simulink model "Aula02_ex01"  (Simulink 7.7)
settings: Solver=VariableStepDiscrete  StartTime=0.0  StopTime=0.006  RelTol=1e-3
settings Model: Creator=Andréa  LastModifiedBy=Andréa
settings SimEventsCC: propDiagAttribOutput=1  propDiagFcnCallOutput=1  propDiagStatOutput=0

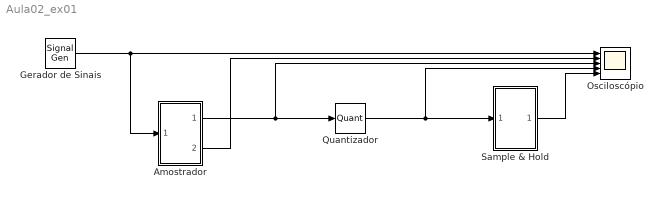
== system Aula02_ex01 ==
  Amostrador : Subsystem
  Gerador de Sinais : SignalGenerator  Frequency=500
  Osciloscópio : Scope  NumInputPorts=5
      settings: YMin=-1~-1~-1~-1~-1  YMax=1~1~1~1~1  SampleInput=on  SampleTime=0.00000001
  Quantizador : Quantizer  QuantizationInterval=0.25
  Sample & Hold : Subsystem
  wires:
  Gerador de Sinais/1 -> Osciloscópio/1, Amostrador/1(In1)
  Amostrador/1(Out1) -> Quantizador/1, Osciloscópio/3
  Quantizador/1 -> Sample & Hold/1(In1), Osciloscópio/4
  Sample & Hold/1(Out1) -> Osciloscópio/5
  Amostrador/2(Out2) -> Osciloscópio/2

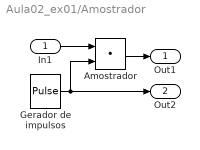
== system Aula02_ex01/Amostrador ==
  In1 : Inport
  Amostrador : DotProduct  InputSameDT=on  OutDataTypeStr=Inherit: Inherit via internal rule
  Gerador de impulsos : DiscretePulseGenerator  PulseType=Time based  Period=1.25e-4
  Out1 : Outport
  Out2 : Outport  Port=2
  wires:
  Gerador de impulsos/1 -> Out2/1, Amostrador/2
  In1/1 -> Amostrador/1
  Amostrador/1 -> Out1/1

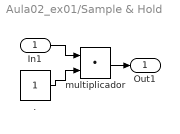
== system Aula02_ex01/Sample & Hold ==
  In1 : Inport
  . : Constant
  multiplicador : DotProduct  SampleTime=1.25e-4  InputSameDT=on  OutDataTypeStr=Inherit: Inherit via internal rule
  Out1 : Outport
  wires:
  In1/1 -> multiplicador/1
  multiplicador/1 -> Out1/1
  ./1 -> multiplicador/2
